simulink model "AbstractTwoVehicleModel"  (R2019b)
settings: Solver=VariableStepAuto  StartTime=0.0  StopTime=50  RelTol=1e-3
model workspace (MAT data in the model file):
  DOWN_TABLE = Simulink.Parameter
  DOWN_TABLE.Value = [0  2.2352  8.9408  15.6464; 0  2.2352  8.9408  15.6464; 0  2.2352  11.176  17.8816; 0  2.2352  13.4112  22.352; 0  13.4112  22.352  35.7632; 0  13.4112  22.352  35.7632]
  DOWN_TABLE.DataType = 'auto'
  DOWN_TABLE.Dimensions = [6 4]
  DOWN_TH_BP = Simulink.Parameter
  DOWN_TH_BP.Value = [0; 25; 35; 50; 90; 100]
  DOWN_TH_BP.DataType = 'auto'
  DOWN_TH_BP.Dimensions = [6 1]
  TWAIT = Simulink.Parameter
  TWAIT.Value = 2
  TWAIT.DataType = 'auto'
  TWAIT.Dimensions = [1 1]
  UP_TABLE = Simulink.Parameter
  UP_TABLE.Value = [4.4704  13.4112  22.352  447040; 4.4704  13.4112  22.352  447040; 6.7056  13.4112  22.352  447040; 10.28192  18.32864  26.8224  447040; 17.8816  31.2928  44.704  447040; 17.8816  31.2928  44.704  447040]
  UP_TABLE.DataType = 'auto'
  UP_TABLE.Dimensions = [6 4]
  UP_TH_BP = Simulink.Parameter
  UP_TH_BP.Value = [0; 25; 35; 50; 90; 100]
  UP_TH_BP.DataType = 'auto'
  UP_TH_BP.Dimensions = [6 1]
libraries: simulink x2, mpcadaslib x2
settings Model: Creator=qihan  LastModifiedBy=mustafa
settings SolverCC: ZeroCrossControl=DisableAll  ZeroCrossAlgorithm=Adaptive  DecoupledContinuousIntegration=on
settings DataIOCC: ReturnWorkspaceOutputsName=tpef60d72c_44c7_4a69_b2c5_cdb6ae33fc37
settings DebuggingCC: IgnoredZcDiagnostic=none
settings SFSimCC: CustomCodeUndefinedFunction=UseInterfaceOnly

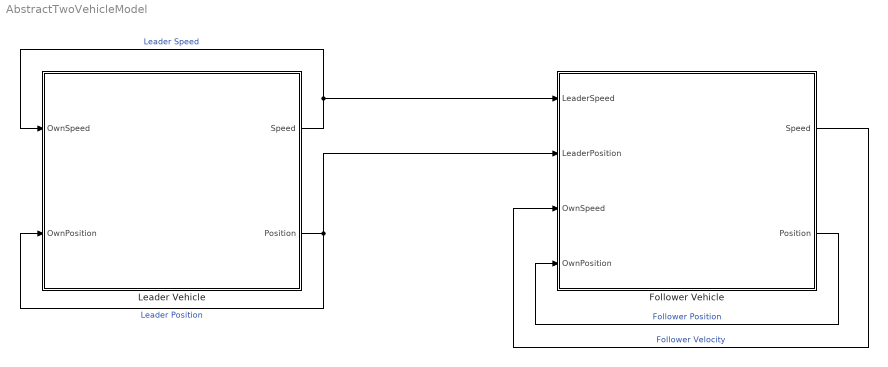
== system AbstractTwoVehicleModel ==
  Follower Vehicle : Subsystem  mask{InitPosition=0, FreeDriveSpeed=35, InitSpeed=45}
      mask prompts: InitPosition "Initial Position"; FreeDriveSpeed "FreeDrive Speed"; InitSpeed "Initial Speed"
      mask TypeOptions InitPosition: initial position/Value
      mask TypeOptions InitSpeed: initial Speed/Value
  Leader Vehicle : Subsystem  mask{InitPosition=100, FreeDriveSpeed=30, InitSpeed=30}
      mask prompts: InitPosition "Initial Position"; FreeDriveSpeed "FreeDrive Speed"; InitSpeed "Initial Speed"
      mask TypeOptions InitPosition: initial position/Value
      mask TypeOptions InitSpeed: initial Speed/Value
  wires:
  Leader Vehicle/1(Speed) -> Leader Vehicle/1(OwnSpeed), Follower Vehicle/1(LeaderSpeed)  "Leader Speed"
  Leader Vehicle/2(Position) -> Leader Vehicle/2(OwnPosition), Follower Vehicle/2(LeaderPosition)  "Leader Position"
  Follower Vehicle/1(Speed) -> Follower Vehicle/3(OwnSpeed)  "Follower Velocity"
  Follower Vehicle/2(Position) -> Follower Vehicle/4(OwnPosition)  "Follower Position"

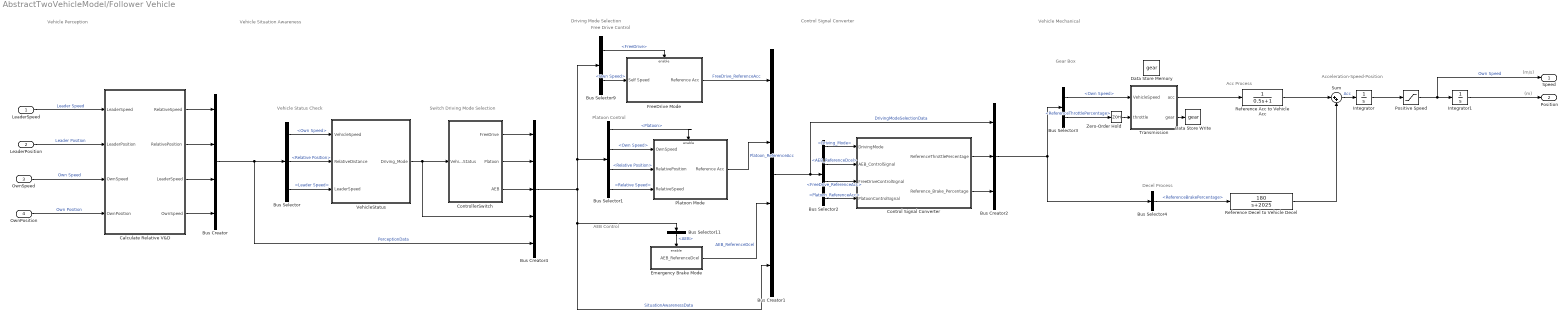
== system AbstractTwoVehicleModel/Follower Vehicle ==
  note: Acceleration-Speed-Position
  note: Vehicle Situation Awareness
  note: Driving Mode Selection
  note: Vehicle Mechanical
  note: AEB Control
  note: Free Drive Control
  note: Platoon Control
  note: Vehicle Status Check
  note: Acc Process
  note: (m)
  note: (m/s)
  note: Decel Process
  note: Vehicle Perception
  note: Switch Driving Mode Selection
  note: Control Signal Converter
  note: Gear Box
  LeaderSpeed : Inport
  LeaderPosition : Inport  Port=2
  OwnSpeed : Inport  Port=3
  OwnPosition : Inport  Port=4
  Bus Creator : BusCreator  Inputs=4
  Bus Creator1 : BusCreator  Inputs=4
  Bus Creator2 : BusCreator  Inputs=3
  Bus Creator4 : BusCreator  Inputs=5
  Bus Selector : BusSelector  OutputSignals=Own Speed,Relative Position,Leader Speed
  Bus Selector1 : BusSelector  OutputSignals=Platoon,PerceptionData.Own Speed,PerceptionData.Relative Position,PerceptionData.Relative Speed
  Bus Selector11 : BusSelector  OutputSignals=AEB
  Bus Selector2 : BusSelector  OutputSignals=SituationAwarenessData.Driving_Mode,AEB_ReferenceDcel,FreeDrive_ReferenceAcc,Platoon_ReferenceAcc
  Bus Selector3 : BusSelector  OutputSignals=DrivingModeSelectionData.SituationAwarenessData.PerceptionData.Own Speed,ReferenceThrottlePercentage
  Bus Selector4 : BusSelector  OutputSignals=ReferenceBrakePercentage
  Bus Selector9 : BusSelector  OutputSignals=FreeDrive,PerceptionData.Own Speed
  Calculate Relative V&D : Subsystem
  Control Signal Converter : Subsystem
  ControllerSwitch : Stateflow chart  BlockKeywords=__PRM__SERIALIZED__DATA__:Stateflow Chart,Stateflow Diagram  TreatAsAtomicUnit=on
  Data Store Memory : DataStoreMemory  DataStoreName=gear  ReadBeforeWriteMsg=warning  WriteAfterWriteMsg=warning  WriteAfterReadMsg=warning  ShowAdditionalParam=off
  Data Store Write : DataStoreWrite  DataStoreName=gear
  Emergency Brake Mode : Subsystem  TreatAsAtomicUnit=on
  FreeDrive Mode : Subsystem  TreatAsAtomicUnit=on
  Integrator : Integrator  InitialCondition=InitSpeed
  Integrator1 : Integrator  InitialCondition=InitPosition
  Platoon Mode : Subsystem  TreatAsAtomicUnit=on
  Positive Speed : Saturate  UpperLimit=inf  LowerLimit=0
  Reference Acc to Vehicle Acc : TransferFcn  Denominator=[0.5 1]
  Reference Decel to Vehicle Decel : TransferFcn  Numerator=[180]  Denominator=[1 2025]
  Sum : Sum  Inputs=|++
  Transmission : Stateflow chart  BlockKeywords=__PRM__SERIALIZED__DATA__:Stateflow Chart,Stateflow Diagram  TreatAsAtomicUnit=on
  VehicleStatus : Stateflow chart  BlockKeywords=__PRM__SERIALIZED__DATA__:Stateflow Chart,Stateflow Diagram  TreatAsAtomicUnit=on
  Zero-Order Hold : ZeroOrderHold  SampleTime=-1
  Speed : Outport  VectorParamsAs1DForOutWhenUnconnected=off
  Position : Outport  Port=2  VectorParamsAs1DForOutWhenUnconnected=off
  wires:
  Reference Acc to Vehicle Acc/1 -> Sum/1
  Reference Decel to Vehicle Decel/1 -> Sum/2
  Sum/1 -> Integrator/1  "Acc"
  Bus Selector/2 -> VehicleStatus/2(RelativeDistance)  "<Relative Position>"
  Integrator/1 -> Positive Speed/1
  Bus Selector/1 -> VehicleStatus/1(VehicleSpeed)  "<Own Speed>"
  Transmission/1(acc) -> Reference Acc to Vehicle Acc/1
  Bus Selector/3 -> VehicleStatus/3(LeaderSpeed)  "<Leader Speed>"
  FreeDrive Mode/1(Reference Acc) -> Bus Creator1/1  "FreeDrive_ReferenceAcc"
  Platoon Mode/1(Reference Acc) -> Bus Creator1/2  "Platoon_ReferenceAcc"
  Emergency Brake Mode/1(AEB_ReferenceDcel) -> Bus Creator1/3  "AEB_ReferenceDcel"
  Positive Speed/1 -> Speed/1, Integrator1/1  "Own Speed"
  Integrator1/1 -> Position/1
  LeaderSpeed/1 -> Calculate Relative V&D/1(LeaderSpeed)  "Leader Speed"
  LeaderPosition/1 -> Calculate Relative V&D/2(LeaderPosition)  "Leader Position"
  Bus Selector9/2 -> FreeDrive Mode/1(Self Speed)  "<Own Speed>"
  Bus Selector9/1 -> FreeDrive Mode/Enable  "<FreeDrive>"
  Bus Selector11/1 -> Emergency Brake Mode/Enable  "<AEB>"
  OwnSpeed/1 -> Calculate Relative V&D/3(OwnSpeed)  "Own Speed"
  OwnPosition/1 -> Calculate Relative V&D/4(OwnPosition)  "Own Position"
  VehicleStatus/1(Driving_Mode) -> Bus Creator4/4, ControllerSwitch/1(Vehicle_Status)
  Transmission/2(gear) -> Data Store Write/1
  Calculate Relative V&D/2(RelativePosition) -> Bus Creator/2
  Calculate Relative V&D/1(RelativeSpeed) -> Bus Creator/1
  Calculate Relative V&D/3("LeaderSpeed ") -> Bus Creator/3
  Calculate Relative V&D/4("OwnSpeed ") -> Bus Creator/4
  Bus Creator/1 -> Bus Creator4/5, Bus Selector/1  "PerceptionData"
  ControllerSwitch/1(FreeDrive) -> Bus Creator4/1
  ControllerSwitch/2(Platoon) -> Bus Creator4/2
  ControllerSwitch/3(AEB) -> Bus Creator4/3
  Bus Creator4/1 -> Bus Selector9/1, Bus Selector1/1, Bus Creator1/4, Bus Selector11/1  "SituationAwarenessData"
  Bus Selector1/1 -> Platoon Mode/Enable  "<Platoon>"
  Bus Selector1/2 -> Platoon Mode/1(OwnSpeed)  "<Own Speed>"
  Bus Selector1/3 -> Platoon Mode/2(RelativePosition)  "<Relative Position>"
  Bus Selector1/4 -> Platoon Mode/3(RelativeSpeed)  "<Relative Speed>"
  Bus Creator1/1 -> Bus Creator2/1, Bus Selector2/1  "DrivingModeSelectionData"
  Bus Selector2/1 -> Control Signal Converter/1(DrivingMode)  "<Driving_Mode>"
  Bus Selector2/2 -> Control Signal Converter/2(AEB_ControlSignal)  "<AEB_ReferenceDcel>"
  Bus Selector2/3 -> Control Signal Converter/3(FreeDriveControlSignal)  "<FreeDrive_ReferenceAcc>"
  Bus Selector2/4 -> Control Signal Converter/4(PlatoonControlSignal)  "<Platoon_ReferenceAcc>"
  Control Signal Converter/1(ReferenceThrottlePercentage) -> Bus Creator2/2
  Control Signal Converter/2(Reference_Brake_Percentage) -> Bus Creator2/3
  Bus Creator2/1 -> Bus Selector4/1, Bus Selector3/1
  Bus Selector3/1 -> Transmission/1(VehicleSpeed)  "<Own Speed>"
  Bus Selector3/2 -> Zero-Order Hold/1  "<ReferenceThrottlePercentage>"
  Bus Selector4/1 -> Reference Decel to Vehicle Decel/1  "<ReferenceBrakePercentage>"
  Zero-Order Hold/1 -> Transmission/2(throttle)

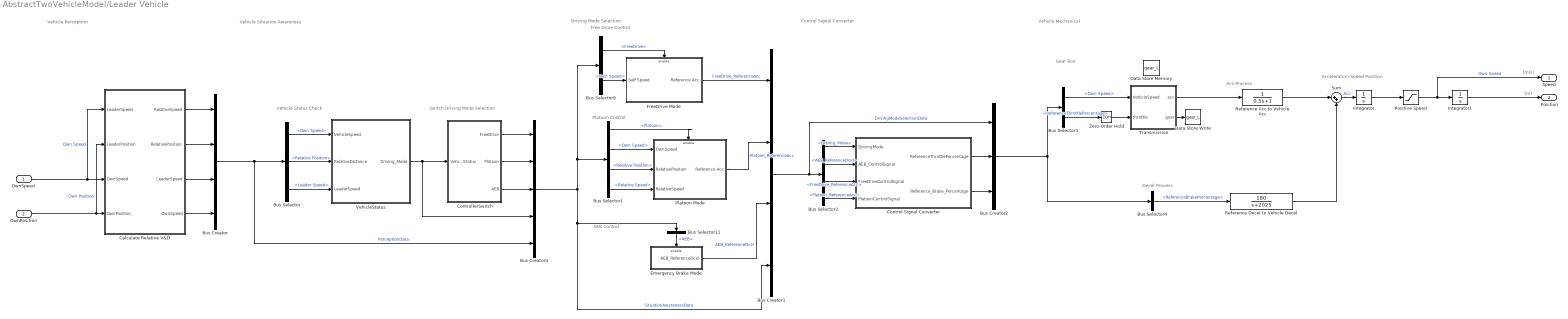
== system AbstractTwoVehicleModel/Leader Vehicle ==
  note: Acceleration-Speed-Position
  note: Vehicle Situation Awareness
  note: Driving Mode Selection
  note: Vehicle Mechanical
  note: AEB Control
  note: Free Drive Control
  note: Platoon Control
  note: Vehicle Status Check
  note: Acc Process
  note: (m)
  note: (m/s)
  note: Decel Process
  note: Vehicle Perception
  note: Switch Driving Mode Selection
  note: Control Signal Converter
  note: Gear Box
  OwnSpeed : Inport
  OwnPosition : Inport  Port=2
  Bus Creator : BusCreator  Inputs=4
  Bus Creator1 : BusCreator  Inputs=4
  Bus Creator2 : BusCreator  Inputs=3
  Bus Creator4 : BusCreator  Inputs=5
  Bus Selector : BusSelector  OutputSignals=Own Speed,Relative Position,Leader Speed
  Bus Selector1 : BusSelector  OutputSignals=Platoon,PerceptionData.Own Speed,PerceptionData.Relative Position,PerceptionData.Relative Speed
  Bus Selector11 : BusSelector  OutputSignals=AEB
  Bus Selector2 : BusSelector  OutputSignals=SituationAwarenessData.Driving_Mode,AEB_ReferenceDcel,FreeDrive_ReferenceAcc,Platoon_ReferenceAcc
  Bus Selector3 : BusSelector  OutputSignals=DrivingModeSelectionData.SituationAwarenessData.PerceptionData.Own Speed,ReferenceThrottlePercentage
  Bus Selector4 : BusSelector  OutputSignals=ReferenceBrakePercentage
  Bus Selector9 : BusSelector  OutputSignals=FreeDrive,PerceptionData.Own Speed
  Calculate Relative V&D : Subsystem
  Control Signal Converter : Subsystem
  ControllerSwitch : Stateflow chart  BlockKeywords=__PRM__SERIALIZED__DATA__:Stateflow Chart,Stateflow Diagram  TreatAsAtomicUnit=on
  Data Store Memory : DataStoreMemory  DataStoreName=gear_L  ReadBeforeWriteMsg=warning  WriteAfterWriteMsg=warning  WriteAfterReadMsg=warning  ShowAdditionalParam=off
  Data Store Write : DataStoreWrite  DataStoreName=gear_L
  Emergency Brake Mode : Subsystem  TreatAsAtomicUnit=on
  FreeDrive Mode : Subsystem  TreatAsAtomicUnit=on
  Integrator : Integrator  InitialCondition=InitSpeed
  Integrator1 : Integrator  InitialCondition=InitPosition
  Platoon Mode : Subsystem  TreatAsAtomicUnit=on
  Positive Speed : Saturate  UpperLimit=inf  LowerLimit=0
  Reference Acc to Vehicle Acc : TransferFcn  Denominator=[0.5 1]
  Reference Decel to Vehicle Decel : TransferFcn  Numerator=[180]  Denominator=[1 2025]
  Sum : Sum  Inputs=|++
  Transmission : Stateflow chart  BlockKeywords=__PRM__SERIALIZED__DATA__:Stateflow Chart,Stateflow Diagram  TreatAsAtomicUnit=on
  VehicleStatus : Stateflow chart  BlockKeywords=__PRM__SERIALIZED__DATA__:Stateflow Chart,Stateflow Diagram  TreatAsAtomicUnit=on
  Zero-Order Hold : ZeroOrderHold  SampleTime=-1
  Speed : Outport  VectorParamsAs1DForOutWhenUnconnected=off
  Position : Outport  Port=2  VectorParamsAs1DForOutWhenUnconnected=off
  wires:
  Reference Acc to Vehicle Acc/1 -> Sum/1
  Reference Decel to Vehicle Decel/1 -> Sum/2
  Sum/1 -> Integrator/1  "Acc"
  Bus Selector/2 -> VehicleStatus/2(RelativeDistance)  "<Relative Position>"
  Integrator/1 -> Positive Speed/1
  Bus Selector/1 -> VehicleStatus/1(VehicleSpeed)  "<Own Speed>"
  Transmission/1(acc) -> Reference Acc to Vehicle Acc/1
  Bus Selector/3 -> VehicleStatus/3(LeaderSpeed)  "<Leader Speed>"
  FreeDrive Mode/1(Reference Acc) -> Bus Creator1/1  "FreeDrive_ReferenceAcc"
  Platoon Mode/1(Reference Acc) -> Bus Creator1/2  "Platoon_ReferenceAcc"
  Emergency Brake Mode/1(AEB_ReferenceDcel) -> Bus Creator1/3  "AEB_ReferenceDcel"
  Positive Speed/1 -> Speed/1, Integrator1/1  "Own Speed"
  Integrator1/1 -> Position/1
  Bus Selector9/2 -> FreeDrive Mode/1(Self Speed)  "<Own Speed>"
  Bus Selector9/1 -> FreeDrive Mode/Enable  "<FreeDrive>"
  Bus Selector11/1 -> Emergency Brake Mode/Enable  "<AEB>"
  OwnSpeed/1 -> Calculate Relative V&D/1(LeaderSpeed), Calculate Relative V&D/3(OwnSpeed)  "Own Speed"
  OwnPosition/1 -> Calculate Relative V&D/2(LeaderPosition), Calculate Relative V&D/4(OwnPosition)  "Own Position"
  VehicleStatus/1(Driving_Mode) -> Bus Creator4/4, ControllerSwitch/1(Vehicle_Status)
  Transmission/2(gear) -> Data Store Write/1
  Calculate Relative V&D/2(RelativePosition) -> Bus Creator/2
  Calculate Relative V&D/1(RelativeSpeed) -> Bus Creator/1
  Calculate Relative V&D/3("LeaderSpeed ") -> Bus Creator/3
  Calculate Relative V&D/4("OwnSpeed ") -> Bus Creator/4
  Bus Creator/1 -> Bus Creator4/5, Bus Selector/1  "PerceptionData"
  ControllerSwitch/1(FreeDrive) -> Bus Creator4/1
  ControllerSwitch/2(Platoon) -> Bus Creator4/2
  ControllerSwitch/3(AEB) -> Bus Creator4/3
  Bus Creator4/1 -> Bus Selector9/1, Bus Selector1/1, Bus Creator1/4, Bus Selector11/1  "SituationAwarenessData"
  Bus Selector1/1 -> Platoon Mode/Enable  "<Platoon>"
  Bus Selector1/2 -> Platoon Mode/1(OwnSpeed)  "<Own Speed>"
  Bus Selector1/3 -> Platoon Mode/2(RelativePosition)  "<Relative Position>"
  Bus Selector1/4 -> Platoon Mode/3(RelativeSpeed)  "<Relative Speed>"
  Bus Creator1/1 -> Bus Creator2/1, Bus Selector2/1  "DrivingModeSelectionData"
  Bus Selector2/1 -> Control Signal Converter/1(DrivingMode)  "<Driving_Mode>"
  Bus Selector2/2 -> Control Signal Converter/2(AEB_ControlSignal)  "<AEB_ReferenceDcel>"
  Bus Selector2/3 -> Control Signal Converter/3(FreeDriveControlSignal)  "<FreeDrive_ReferenceAcc>"
  Bus Selector2/4 -> Control Signal Converter/4(PlatoonControlSignal)  "<Platoon_ReferenceAcc>"
  Control Signal Converter/1(ReferenceThrottlePercentage) -> Bus Creator2/2
  Control Signal Converter/2(Reference_Brake_Percentage) -> Bus Creator2/3
  Bus Creator2/1 -> Bus Selector4/1, Bus Selector3/1
  Bus Selector3/1 -> Transmission/1(VehicleSpeed)  "<Own Speed>"
  Bus Selector3/2 -> Zero-Order Hold/1  "<ReferenceThrottlePercentage>"
  Bus Selector4/1 -> Reference Decel to Vehicle Decel/1  "<ReferenceBrakePercentage>"
  Zero-Order Hold/1 -> Transmission/2(throttle)

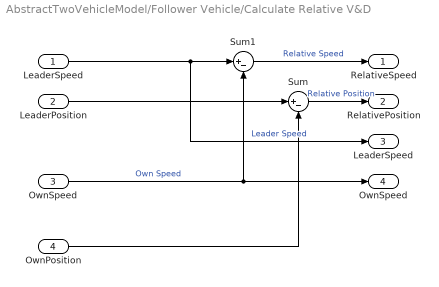
== system AbstractTwoVehicleModel/Follower Vehicle/Calculate Relative V&D ==
  LeaderSpeed : Inport
  LeaderPosition : Inport  Port=2
  OwnSpeed : Inport  Port=3
  OwnPosition : Inport  Port=4
  Sum : Sum  Inputs=|+-
  Sum1 : Sum  Inputs=|+-
  RelativeSpeed : Outport  VectorParamsAs1DForOutWhenUnconnected=off
  RelativePosition : Outport  Port=2  VectorParamsAs1DForOutWhenUnconnected=off
  "LeaderSpeed " : Outport  Port=3  VectorParamsAs1DForOutWhenUnconnected=off
  "OwnSpeed " : Outport  Port=4  VectorParamsAs1DForOutWhenUnconnected=off
  wires:
  Sum/1 -> RelativePosition/1  "Relative Position"
  LeaderPosition/1 -> Sum/1
  LeaderSpeed/1 -> "LeaderSpeed "/1, Sum1/1  "Leader Speed"
  OwnPosition/1 -> Sum/2
  Sum1/1 -> RelativeSpeed/1  "Relative Speed"
  OwnSpeed/1 -> "OwnSpeed "/1, Sum1/2  "Own Speed"

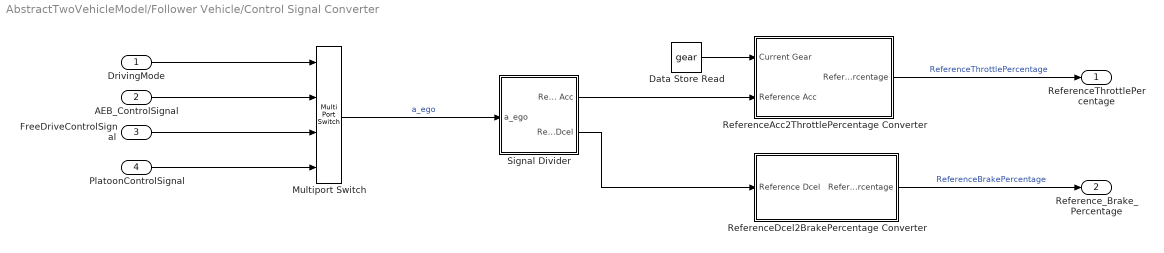
== system AbstractTwoVehicleModel/Follower Vehicle/Control Signal Converter ==
  DrivingMode : Inport
  AEB_ControlSignal : Inport  Port=2
  FreeDriveControlSignal : Inport  Port=3
  PlatoonControlSignal : Inport  Port=4
  Data Store Read : DataStoreRead  DataStoreName=gear
  Multiport Switch : MultiPortSwitch  DiagnosticForDefault=None
  ReferenceAcc2ThrottlePercentage Converter : Subsystem
  ReferenceDcel2BrakePercentage Converter : Subsystem
  Signal Divider : Subsystem
  ReferenceThrottlePercentage : Outport  VectorParamsAs1DForOutWhenUnconnected=off
  Reference_Brake_Percentage : Outport  Port=2  VectorParamsAs1DForOutWhenUnconnected=off
  wires:
  Signal Divider/1(Reference Acc) -> ReferenceAcc2ThrottlePercentage Converter/2(Reference Acc)
  ReferenceDcel2BrakePercentage Converter/1(Reference Brake Percentage) -> Reference_Brake_Percentage/1  "ReferenceBrakePercentage"
  Signal Divider/2(Reference Dcel) -> ReferenceDcel2BrakePercentage Converter/1(Reference Dcel)
  Multiport Switch/1 -> Signal Divider/1(a_ego)  "a_ego"
  Data Store Read/1 -> ReferenceAcc2ThrottlePercentage Converter/1(Current Gear)
  ReferenceAcc2ThrottlePercentage Converter/1(Reference Throttle Percentage) -> ReferenceThrottlePercentage/1  "ReferenceThrottlePercentage"
  DrivingMode/1 -> Multiport Switch/1
  AEB_ControlSignal/1 -> Multiport Switch/2
  FreeDriveControlSignal/1 -> Multiport Switch/3
  PlatoonControlSignal/1 -> Multiport Switch/4

== system AbstractTwoVehicleModel/Follower Vehicle/Emergency Brake Mode ==
  Enable : EnablePort
  Constant : Constant  Value=-10
  AEB_ReferenceDcel : Outport  OutputWhenDisabled=reset  InitialOutput=[0]  VectorParamsAs1DForOutWhenUnconnected=off
  wires:
  Constant/1 -> AEB_ReferenceDcel/1

== system AbstractTwoVehicleModel/Follower Vehicle/FreeDrive Mode ==
  Self Speed : Inport
  Enable : EnablePort  StatesWhenEnabling=reset
  FreeDrive Speed : Constant  Value=FreeDriveSpeed
  PID Controller1 : simulink/Continuous/PID Controller  Controller=PI  Form=Parallel  TimeDomain=Continuous-time  SampleTime=-1  IntegratorMethod=Forward Euler  FilterMethod=Forward Euler  ControllerParametersSource=internal  P=2.0341199375219  I=0.0356576460366845  D=2.08363010404189  UseFilter=on  N=233.214579742572  TunerSelectOption=Transfer Function Based (PID Tuner App)  ZeroCross=off  InitialConditionSource=internal  InitialConditionForIntegrator=0  InitialConditionForFilter=0  DifferentiatorICPrevScaledInput=0  ExternalReset=none  IgnoreLimit=on  TrackingMode=off  Kt=1  LimitOutput=on  UpperSaturationLimit=2  LowerSaturationLimit=-2  LinearizeAsGain=on  AntiWindupMode=clamping  Kb=1  POutMin=[]  POutMax=[]  IOutMin=[]  IOutMax=[]  DOutMin=[]  DOutMax=[]  NOutMin=[]  NOutMax=[]  SumOutMin=[]  SumOutMax=[]  SaturationOutMin=[]  SaturationOutMax=[]  PParamMin=[]  PParamMax=[]  IParamMin=[]  IParamMax=[]  DParamMin=[]  DParamMax=[]  NParamMin=[]  NParamMax=[]  KbParamMin=[]  KbParamMax=[]  KtParamMin=[]  KtParamMax=[]  KbOutMin=[]  KbOutMax=[]  KtOutMin=[]  KtOutMax=[]  IntegratorOutMin=[]  IntegratorOutMax=[]  FilterOutMin=[]  FilterOutMax=[]  SumI1OutMin=[]  SumI1OutMax=[]  SumI2OutMin=[]  SumI2OutMax=[]  SumI3OutMin=[]  SumI3OutMax=[]  SumI4OutMin=[]  SumI4OutMax=[]  SumDOutMin=[]  SumDOutMax=[]  DifferentiatorOutMin=[]  DifferentiatorOutMax=[]  FilterDiffOutCoefMin=[]  FilterDiffOutCoefMax=[]  ReciprocalOutMin=[]  ReciprocalOutMax=[]  SumDenOutMin=[]  SumDenOutMax=[]  SumNumOutMin=[]  SumNumOutMax=[]  DivideOutMin=[]  DivideOutMax=[]  IntegratorContinuousStateAttributes=''  IntegratorStateMustResolveToSignalObject=off  IntegratorRTWStateStorageClass=Auto  FilterContinuousStateAttributes=''  FilterStateMustResolveToSignalObject=off  FilterRTWStateStorageClass=Auto  ParallelPVariant=InternalParameters  IdealPVariant=Disabled  IVariant=InternalParameters  DVariant=Disabled  IntegratorVariant=Continuous  SatVariant=Enabled  AWVariant=ContClampingParallel  PCopyVariant=Disabled  TRVariant=Disabled  FdbkBlocksVariant=Forward  IdealPFdbkVariant=Disabled  SatFdbkVariant=Disabled  DerivativeFilterVariant=Disabled  NVariant=Disabled  NCopyVariant=Disabled_SignalSpec  FilterICVariant=Disabled  IntegratorICVariant=InternalICs  ExternalResetVariant=Disabled  TRSumVariant=Passthrough  SumFdbkVariant=Disabled  SumVariant=Sum_PI
  Sum16 : Sum  Inputs=|+-
  Reference Acc : Outport  OutputWhenDisabled=reset  InitialOutput=[0]  VectorParamsAs1DForOutWhenUnconnected=off
  wires:
  Self Speed/1 -> Sum16/2
  FreeDrive Speed/1 -> Sum16/1
  Sum16/1 -> PID Controller1/1
  PID Controller1/1 -> Reference Acc/1

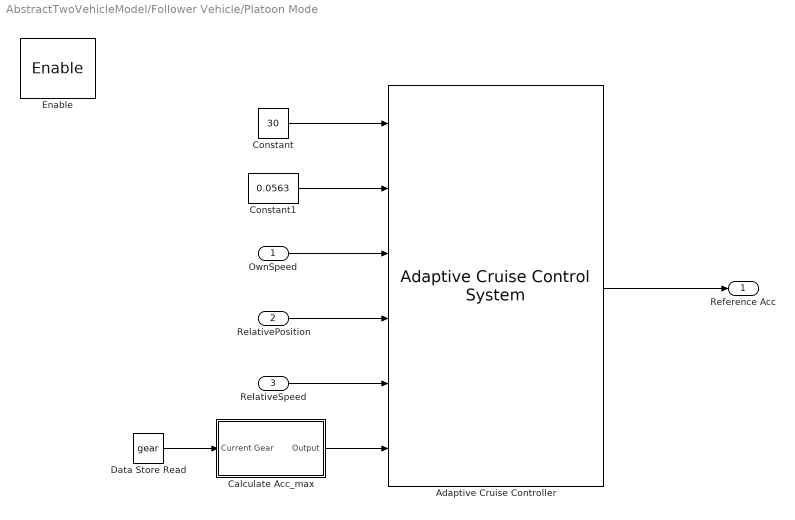
== system AbstractTwoVehicleModel/Follower Vehicle/Platoon Mode ==
  OwnSpeed : Inport
  RelativePosition : Inport  Port=2
  RelativeSpeed : Inport  Port=3
  Enable : EnablePort  StatesWhenEnabling=reset
  Adaptive Cruise Controller : mpcadaslib/Adaptive Cruise Control System  EgoModel=tf(1,[0.5,1,0])  InitialEgoVelocity=20  DefaultSpacing=10  MaxVelocity=50  MinAcceleration=-2  amin_ext=off  MaxAcceleration=2  amax_ext=on  Ts=0.1  PredictionHorizon=30  ControllerBehavior=0.260  suboptimal=off  maxiter=10  datatypeopt=double  optmode=off  trackmode=off
      settings: SourceProductName=Model Predictive Control Toolbox
  Calculate Acc_max : Subsystem
  Constant : Constant  Value=30
  Constant1 : Constant  Value=0.0563
  Data Store Read : DataStoreRead  DataStoreName=gear
  Reference Acc : Outport  OutputWhenDisabled=reset  InitialOutput=[0]  VectorParamsAs1DForOutWhenUnconnected=off
  wires:
  Constant/1 -> Adaptive Cruise Controller/1
  OwnSpeed/1 -> Adaptive Cruise Controller/3
  RelativePosition/1 -> Adaptive Cruise Controller/4
  RelativeSpeed/1 -> Adaptive Cruise Controller/5
  Adaptive Cruise Controller/1 -> Reference Acc/1
  Data Store Read/1 -> Calculate Acc_max/1(Current Gear)
  Calculate Acc_max/1(Output) -> Adaptive Cruise Controller/6
  Constant1/1 -> Adaptive Cruise Controller/2

== system AbstractTwoVehicleModel/Follower Vehicle/Transmission/ComputeThreshold ==
  note: Threshold Calculation
  gear : Inport  OutDataTypeStr=double  PortDimensions=1
  throttle : Inport  Port=2  OutDataTypeStr=double  PortDimensions=1
  f : TriggerPort  TriggerType=function-call  VariantControl=(inherit)
      settings: CopyFcn=Stateflow.SLINSF.SimulinkMan.removeBlockPreDeleteFcn  PreDeleteFcn=Stateflow.SLINSF.SimulinkMan.unsafePredeleteFcn
  InterpDown : Lookup_n-D  BreakpointsForDimension1=DOWN_TH_BP  BreakpointsForDimension2=[1:4]  Table=DOWN_TABLE  OutDataTypeStr=double  LockScale=on
  InterpUp : Lookup_n-D  BreakpointsForDimension1=UP_TH_BP  BreakpointsForDimension2=[1:4]  Table=UP_TABLE  OutDataTypeStr=double  LockScale=on
  down_th : Outport  VectorParamsAs1DForOutWhenUnconnected=off
  up_th : Outport  Port=2  VectorParamsAs1DForOutWhenUnconnected=off
  wires:
  throttle/1 -> InterpDown/1, InterpUp/1
  gear/1 -> InterpDown/2, InterpUp/2
  InterpDown/1 -> down_th/1
  InterpUp/1 -> up_th/1

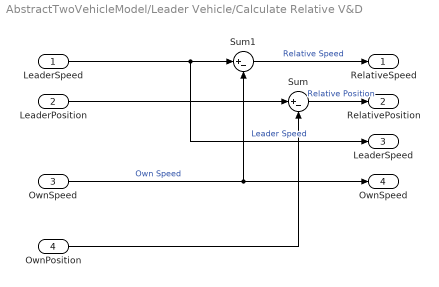
== system AbstractTwoVehicleModel/Leader Vehicle/Calculate Relative V&D ==
  LeaderSpeed : Inport
  LeaderPosition : Inport  Port=2
  OwnSpeed : Inport  Port=3
  OwnPosition : Inport  Port=4
  Sum : Sum  Inputs=|+-
  Sum1 : Sum  Inputs=|+-
  RelativeSpeed : Outport  VectorParamsAs1DForOutWhenUnconnected=off
  RelativePosition : Outport  Port=2  VectorParamsAs1DForOutWhenUnconnected=off
  "LeaderSpeed " : Outport  Port=3  VectorParamsAs1DForOutWhenUnconnected=off
  "OwnSpeed " : Outport  Port=4  VectorParamsAs1DForOutWhenUnconnected=off
  wires:
  Sum/1 -> RelativePosition/1  "Relative Position"
  LeaderPosition/1 -> Sum/1
  LeaderSpeed/1 -> "LeaderSpeed "/1, Sum1/1  "Leader Speed"
  OwnPosition/1 -> Sum/2
  Sum1/1 -> RelativeSpeed/1  "Relative Speed"
  OwnSpeed/1 -> "OwnSpeed "/1, Sum1/2  "Own Speed"

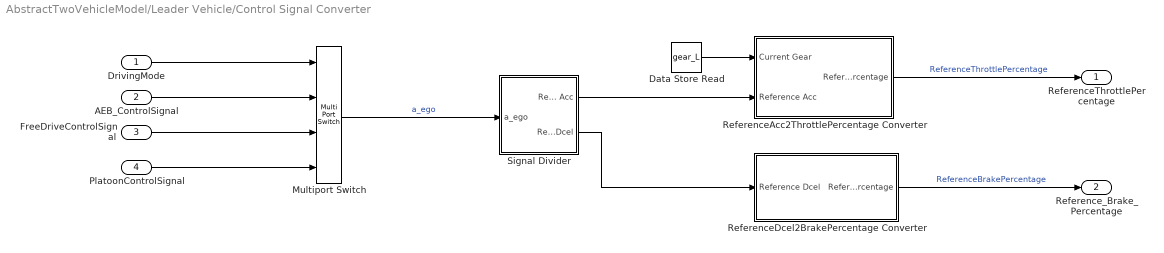
== system AbstractTwoVehicleModel/Leader Vehicle/Control Signal Converter ==
  DrivingMode : Inport
  AEB_ControlSignal : Inport  Port=2
  FreeDriveControlSignal : Inport  Port=3
  PlatoonControlSignal : Inport  Port=4
  Data Store Read : DataStoreRead  DataStoreName=gear_L
  Multiport Switch : MultiPortSwitch  DiagnosticForDefault=None
  ReferenceAcc2ThrottlePercentage Converter : Subsystem
  ReferenceDcel2BrakePercentage Converter : Subsystem
  Signal Divider : Subsystem
  ReferenceThrottlePercentage : Outport  VectorParamsAs1DForOutWhenUnconnected=off
  Reference_Brake_Percentage : Outport  Port=2  VectorParamsAs1DForOutWhenUnconnected=off
  wires:
  Signal Divider/1(Reference Acc) -> ReferenceAcc2ThrottlePercentage Converter/2(Reference Acc)
  ReferenceDcel2BrakePercentage Converter/1(Reference Brake Percentage) -> Reference_Brake_Percentage/1  "ReferenceBrakePercentage"
  Signal Divider/2(Reference Dcel) -> ReferenceDcel2BrakePercentage Converter/1(Reference Dcel)
  Multiport Switch/1 -> Signal Divider/1(a_ego)  "a_ego"
  Data Store Read/1 -> ReferenceAcc2ThrottlePercentage Converter/1(Current Gear)
  ReferenceAcc2ThrottlePercentage Converter/1(Reference Throttle Percentage) -> ReferenceThrottlePercentage/1  "ReferenceThrottlePercentage"
  DrivingMode/1 -> Multiport Switch/1
  AEB_ControlSignal/1 -> Multiport Switch/2
  FreeDriveControlSignal/1 -> Multiport Switch/3
  PlatoonControlSignal/1 -> Multiport Switch/4

== system AbstractTwoVehicleModel/Leader Vehicle/Emergency Brake Mode ==
  Enable : EnablePort
  Constant : Constant  Value=-10
  AEB_ReferenceDcel : Outport  OutputWhenDisabled=reset  InitialOutput=[0]  VectorParamsAs1DForOutWhenUnconnected=off
  wires:
  Constant/1 -> AEB_ReferenceDcel/1

== system AbstractTwoVehicleModel/Leader Vehicle/FreeDrive Mode ==
  Self Speed : Inport
  Enable : EnablePort  StatesWhenEnabling=reset
  FreeDrive Speed : Constant  Value=FreeDriveSpeed
  PID Controller1 : simulink/Continuous/PID Controller  Controller=PI  Form=Parallel  TimeDomain=Continuous-time  SampleTime=-1  IntegratorMethod=Forward Euler  FilterMethod=Forward Euler  ControllerParametersSource=internal  P=2.0341199375219  I=0.0356576460366845  D=2.08363010404189  UseFilter=on  N=233.214579742572  TunerSelectOption=Transfer Function Based (PID Tuner App)  ZeroCross=off  InitialConditionSource=internal  InitialConditionForIntegrator=0  InitialConditionForFilter=0  DifferentiatorICPrevScaledInput=0  ExternalReset=none  TrackingMode=off  Kt=1  LimitOutput=on  UpperSaturationLimit=2  LowerSaturationLimit=-3  LinearizeAsGain=on  AntiWindupMode=clamping  Kb=1  POutMin=[]  POutMax=[]  IOutMin=[]  IOutMax=[]  DOutMin=[]  DOutMax=[]  NOutMin=[]  NOutMax=[]  SumOutMin=[]  SumOutMax=[]  SaturationOutMin=[]  SaturationOutMax=[]  PParamMin=[]  PParamMax=[]  IParamMin=[]  IParamMax=[]  DParamMin=[]  DParamMax=[]  NParamMin=[]  NParamMax=[]  KbParamMin=[]  KbParamMax=[]  KtParamMin=[]  KtParamMax=[]  KbOutMin=[]  KbOutMax=[]  KtOutMin=[]  KtOutMax=[]  IntegratorOutMin=[]  IntegratorOutMax=[]  FilterOutMin=[]  FilterOutMax=[]  SumI1OutMin=[]  SumI1OutMax=[]  SumI2OutMin=[]  SumI2OutMax=[]  SumI3OutMin=[]  SumI3OutMax=[]  SumI4OutMin=[]  SumI4OutMax=[]  SumDOutMin=[]  SumDOutMax=[]  DifferentiatorOutMin=[]  DifferentiatorOutMax=[]  FilterDiffOutCoefMin=[]  FilterDiffOutCoefMax=[]  ReciprocalOutMin=[]  ReciprocalOutMax=[]  SumDenOutMin=[]  SumDenOutMax=[]  SumNumOutMin=[]  SumNumOutMax=[]  DivideOutMin=[]  DivideOutMax=[]  IntegratorContinuousStateAttributes=''  IntegratorStateMustResolveToSignalObject=off  IntegratorRTWStateStorageClass=Auto  FilterContinuousStateAttributes=''  FilterStateMustResolveToSignalObject=off  FilterRTWStateStorageClass=Auto  ParallelPVariant=InternalParameters  IdealPVariant=Disabled  IVariant=InternalParameters  DVariant=Disabled  IntegratorVariant=Continuous  SatVariant=Enabled  AWVariant=ContClampingParallel  PCopyVariant=Disabled  TRVariant=Disabled  FdbkBlocksVariant=Forward  IdealPFdbkVariant=Disabled  SatFdbkVariant=Disabled  DerivativeFilterVariant=Disabled  NVariant=Disabled  NCopyVariant=Disabled_SignalSpec  FilterICVariant=Disabled  IntegratorICVariant=InternalICs  ExternalResetVariant=Disabled  TRSumVariant=Passthrough  SumFdbkVariant=Disabled  SumVariant=Sum_PI
  Sum16 : Sum  Inputs=|+-
  Reference Acc : Outport  OutputWhenDisabled=reset  InitialOutput=[0]  VectorParamsAs1DForOutWhenUnconnected=off
  wires:
  Self Speed/1 -> Sum16/2
  FreeDrive Speed/1 -> Sum16/1
  Sum16/1 -> PID Controller1/1
  PID Controller1/1 -> Reference Acc/1

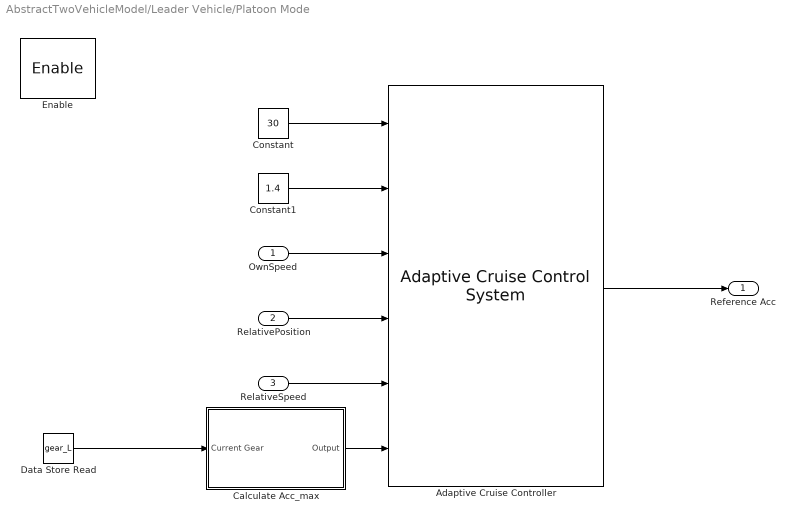
== system AbstractTwoVehicleModel/Leader Vehicle/Platoon Mode ==
  OwnSpeed : Inport
  RelativePosition : Inport  Port=2
  RelativeSpeed : Inport  Port=3
  Enable : EnablePort  StatesWhenEnabling=reset
  Adaptive Cruise Controller : mpcadaslib/Adaptive Cruise Control System  EgoModel=tf(1,[0.5,1,0])  InitialEgoVelocity=20  DefaultSpacing=10  MaxVelocity=50  MinAcceleration=-2  amin_ext=off  MaxAcceleration=2  amax_ext=on  Ts=0.1  PredictionHorizon=30  ControllerBehavior=0.5  suboptimal=off  maxiter=10  datatypeopt=double  optmode=off  trackmode=off
      settings: SourceProductName=Model Predictive Control Toolbox
  Calculate Acc_max : Subsystem
  Constant : Constant  Value=30
  Constant1 : Constant  Value=1.4
  Data Store Read : DataStoreRead  DataStoreName=gear_L
  Reference Acc : Outport  OutputWhenDisabled=reset  InitialOutput=[0]  VectorParamsAs1DForOutWhenUnconnected=off
  wires:
  Constant/1 -> Adaptive Cruise Controller/1
  OwnSpeed/1 -> Adaptive Cruise Controller/3
  RelativePosition/1 -> Adaptive Cruise Controller/4
  RelativeSpeed/1 -> Adaptive Cruise Controller/5
  Adaptive Cruise Controller/1 -> Reference Acc/1
  Constant1/1 -> Adaptive Cruise Controller/2
  Data Store Read/1 -> Calculate Acc_max/1(Current Gear)
  Calculate Acc_max/1(Output) -> Adaptive Cruise Controller/6

== system AbstractTwoVehicleModel/Leader Vehicle/Transmission/ComputeThreshold ==
  note: Threshold Calculation
  gear : Inport  OutDataTypeStr=double  PortDimensions=1
  throttle : Inport  Port=2  OutDataTypeStr=double  PortDimensions=1
  f : TriggerPort  TriggerType=function-call  VariantControl=(inherit)
      settings: CopyFcn=Stateflow.SLINSF.SimulinkMan.removeBlockPreDeleteFcn  PreDeleteFcn=Stateflow.SLINSF.SimulinkMan.unsafePredeleteFcn
  InterpDown : Lookup_n-D  BreakpointsForDimension1=DOWN_TH_BP  BreakpointsForDimension2=[1:4]  Table=DOWN_TABLE  OutDataTypeStr=double  LockScale=on
  InterpUp : Lookup_n-D  BreakpointsForDimension1=UP_TH_BP  BreakpointsForDimension2=[1:4]  Table=UP_TABLE  OutDataTypeStr=double  LockScale=on
  down_th : Outport  VectorParamsAs1DForOutWhenUnconnected=off
  up_th : Outport  Port=2  VectorParamsAs1DForOutWhenUnconnected=off
  wires:
  throttle/1 -> InterpDown/1, InterpUp/1
  gear/1 -> InterpDown/2, InterpUp/2
  InterpDown/1 -> down_th/1
  InterpUp/1 -> up_th/1

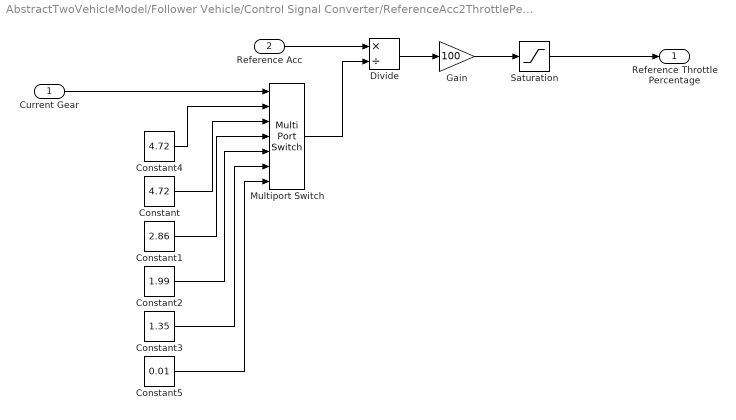
== system AbstractTwoVehicleModel/Follower Vehicle/Control Signal Converter/ReferenceAcc2ThrottlePercentage Converter ==
  Current Gear : Inport
  Reference Acc : Inport  Port=2
  Constant : Constant  Value=4.72
  Constant1 : Constant  Value=2.86
  Constant2 : Constant  Value=1.99
  Constant3 : Constant  Value=1.35
  Constant4 : Constant  Value=4.72
  Constant5 : Constant  Value=0.01
  Divide : Product  Inputs=*/
  Gain : Gain  Gain=100
  Multiport Switch : MultiPortSwitch  DataPortOrder=Zero-based contiguous  Inputs=6  zeroidx=on
  Saturation : Saturate  UpperLimit=100  LowerLimit=0  ZeroCross=off
  Reference Throttle Percentage : Outport  VectorParamsAs1DForOutWhenUnconnected=off
  wires:
  Multiport Switch/1 -> Divide/2
  Constant1/1 -> Multiport Switch/4
  Constant5/1 -> Multiport Switch/7
  Constant3/1 -> Multiport Switch/6
  Reference Acc/1 -> Divide/1
  Constant/1 -> Multiport Switch/3
  Constant4/1 -> Multiport Switch/2
  Constant2/1 -> Multiport Switch/5
  Current Gear/1 -> Multiport Switch/1
  Divide/1 -> Gain/1
  Gain/1 -> Saturation/1
  Saturation/1 -> Reference Throttle Percentage/1

== system AbstractTwoVehicleModel/Follower Vehicle/Control Signal Converter/ReferenceDcel2BrakePercentage Converter ==
  Reference Dcel : Inport
  Constant : Constant  Value=3
  Divide : Product  Inputs=*/
  Gain : Gain  Gain=100
  Saturation : Saturate  UpperLimit=0  LowerLimit=-100
  Reference Brake Percentage : Outport  VectorParamsAs1DForOutWhenUnconnected=off
  wires:
  Reference Dcel/1 -> Divide/1
  Divide/1 -> Gain/1
  Gain/1 -> Saturation/1
  Saturation/1 -> Reference Brake Percentage/1
  Constant/1 -> Divide/2

== system AbstractTwoVehicleModel/Follower Vehicle/Control Signal Converter/Signal Divider ==
  a_ego : Inport
  Constant2 : Constant  Value=0
  Switch : Switch  Criteria=u2 > Threshold
  Switch1 : Switch  Criteria=u2 > Threshold
  Reference Acc : Outport  VectorParamsAs1DForOutWhenUnconnected=off
  Reference Dcel : Outport  Port=2  VectorParamsAs1DForOutWhenUnconnected=off
  wires:
  Constant2/1 -> Switch1/1, Switch/3
  a_ego/1 -> Switch/1, Switch/2, Switch1/2, Switch1/3
  Switch1/1 -> Reference Dcel/1
  Switch/1 -> Reference Acc/1

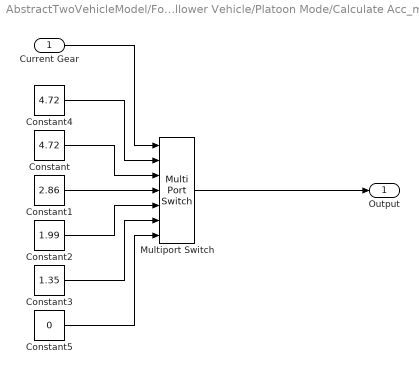
== system AbstractTwoVehicleModel/Follower Vehicle/Platoon Mode/Calculate Acc_max ==
  Current Gear : Inport
  Constant : Constant  Value=4.72
  Constant1 : Constant  Value=2.86
  Constant2 : Constant  Value=1.99
  Constant3 : Constant  Value=1.35
  Constant4 : Constant  Value=4.72
  Constant5 : Constant  Value=0
  Multiport Switch : MultiPortSwitch  DataPortOrder=Zero-based contiguous  Inputs=6  DiagnosticForDefault=None  zeroidx=on
  Output : Outport  VectorParamsAs1DForOutWhenUnconnected=off
  wires:
  Constant1/1 -> Multiport Switch/4
  Constant5/1 -> Multiport Switch/7
  Constant3/1 -> Multiport Switch/6
  Current Gear/1 -> Multiport Switch/1
  Constant/1 -> Multiport Switch/3
  Constant4/1 -> Multiport Switch/2
  Multiport Switch/1 -> Output/1
  Constant2/1 -> Multiport Switch/5

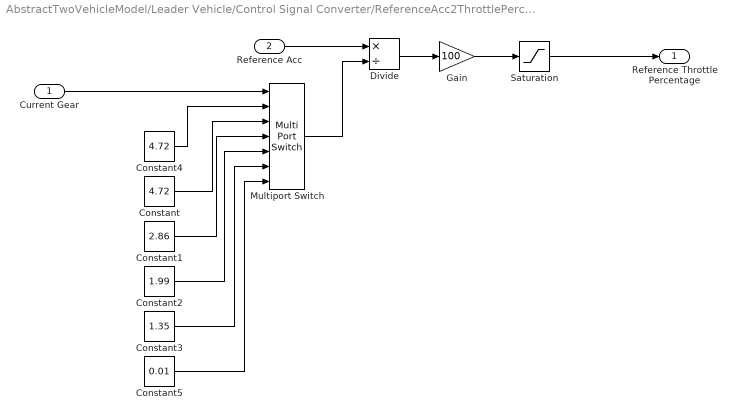
== system AbstractTwoVehicleModel/Leader Vehicle/Control Signal Converter/ReferenceAcc2ThrottlePercentage Converter ==
  Current Gear : Inport
  Reference Acc : Inport  Port=2
  Constant : Constant  Value=4.72
  Constant1 : Constant  Value=2.86
  Constant2 : Constant  Value=1.99
  Constant3 : Constant  Value=1.35
  Constant4 : Constant  Value=4.72
  Constant5 : Constant  Value=0.01
  Divide : Product  Inputs=*/
  Gain : Gain  Gain=100
  Multiport Switch : MultiPortSwitch  DataPortOrder=Zero-based contiguous  Inputs=6  zeroidx=on
  Saturation : Saturate  UpperLimit=100  LowerLimit=0  ZeroCross=off
  Reference Throttle Percentage : Outport  VectorParamsAs1DForOutWhenUnconnected=off
  wires:
  Multiport Switch/1 -> Divide/2
  Constant1/1 -> Multiport Switch/4
  Constant5/1 -> Multiport Switch/7
  Constant3/1 -> Multiport Switch/6
  Reference Acc/1 -> Divide/1
  Constant/1 -> Multiport Switch/3
  Constant4/1 -> Multiport Switch/2
  Constant2/1 -> Multiport Switch/5
  Current Gear/1 -> Multiport Switch/1
  Divide/1 -> Gain/1
  Gain/1 -> Saturation/1
  Saturation/1 -> Reference Throttle Percentage/1

== system AbstractTwoVehicleModel/Leader Vehicle/Control Signal Converter/ReferenceDcel2BrakePercentage Converter ==
  Reference Dcel : Inport
  Constant : Constant  Value=3
  Divide : Product  Inputs=*/
  Gain : Gain  Gain=100
  Saturation : Saturate  UpperLimit=0  LowerLimit=-100
  Reference Brake Percentage : Outport  VectorParamsAs1DForOutWhenUnconnected=off
  wires:
  Reference Dcel/1 -> Divide/1
  Divide/1 -> Gain/1
  Gain/1 -> Saturation/1
  Saturation/1 -> Reference Brake Percentage/1
  Constant/1 -> Divide/2

== system AbstractTwoVehicleModel/Leader Vehicle/Control Signal Converter/Signal Divider ==
  a_ego : Inport
  Constant2 : Constant  Value=0
  Switch : Switch  Criteria=u2 > Threshold
  Switch1 : Switch  Criteria=u2 > Threshold
  Reference Acc : Outport  VectorParamsAs1DForOutWhenUnconnected=off
  Reference Dcel : Outport  Port=2  VectorParamsAs1DForOutWhenUnconnected=off
  wires:
  Constant2/1 -> Switch1/1, Switch/3
  a_ego/1 -> Switch/1, Switch/2, Switch1/2, Switch1/3
  Switch1/1 -> Reference Dcel/1
  Switch/1 -> Reference Acc/1

== system AbstractTwoVehicleModel/Leader Vehicle/Platoon Mode/Calculate Acc_max ==
  Current Gear : Inport
  Constant : Constant  Value=4.72
  Constant1 : Constant  Value=2.86
  Constant2 : Constant  Value=1.99
  Constant3 : Constant  Value=1.35
  Constant4 : Constant  Value=4.72
  Constant5 : Constant  Value=0
  Multiport Switch : MultiPortSwitch  DataPortOrder=Zero-based contiguous  Inputs=6  DiagnosticForDefault=None  zeroidx=on
  Output : Outport  VectorParamsAs1DForOutWhenUnconnected=off
  wires:
  Constant1/1 -> Multiport Switch/4
  Constant5/1 -> Multiport Switch/7
  Constant3/1 -> Multiport Switch/6
  Current Gear/1 -> Multiport Switch/1
  Constant/1 -> Multiport Switch/3
  Constant4/1 -> Multiport Switch/2
  Multiport Switch/1 -> Output/1
  Constant2/1 -> Multiport Switch/5

== stateflow chart AbstractTwoVehicleModel/Leader Vehicle/ControllerSwitch ==
  state Platoon_Controller
    entry:
    Platoon=1;
    FreeDrive=0;
    AEB=0;
  state Choose_Controller
    entry:
    Platoon=0;
    FreeDrive=0;
    AEB=0;
  state FreeDrive_Controller
    entry:
    Platoon=0;
    FreeDrive=1;
    AEB=0;
  state AEB
    entry:
    Platoon=0;
    FreeDrive=0;
    AEB=1;
  (default) -> Choose_Controller
  Choose_Controller -> Platoon_Controller [order 2] : [Vehicle_Status==3]
  FreeDrive_Controller -> Platoon_Controller [order 1] : [Vehicle_Status==3]
  Platoon_Controller -> FreeDrive_Controller [order 2] : [Vehicle_Status==2]
  Platoon_Controller -> AEB [order 1] : [Vehicle_Status==1]
  AEB -> Platoon_Controller [order 2] : [Vehicle_Status==3]
  Choose_Controller -> FreeDrive_Controller [order 1] : [Vehicle_Status==2]
  Choose_Controller -> AEB [order 3] : [Vehicle_Status==1]
  FreeDrive_Controller -> AEB [order 2] : [Vehicle_Status==1]
  AEB -> FreeDrive_Controller [order 1] : [Vehicle_Status==2]
  data: FreeDrive output; Platoon output; Vehicle_Status input; AEB output

== stateflow chart AbstractTwoVehicleModel/Follower Vehicle/ControllerSwitch ==
  state Platoon_Controller
    entry:
    Platoon=1;
    FreeDrive=0;
    AEB=0;
  state Choose_Controller
    entry:
    Platoon=0;
    FreeDrive=0;
    AEB=0;
  state FreeDrive_Controller
    entry:
    Platoon=0;
    FreeDrive=1;
    AEB=0;
  state AEB
    entry:
    Platoon=0;
    FreeDrive=0;
    AEB=1;
  (default) -> Choose_Controller
  Choose_Controller -> Platoon_Controller [order 2] : [Vehicle_Status==3]
  FreeDrive_Controller -> Platoon_Controller [order 1] : [Vehicle_Status==3]
  Platoon_Controller -> FreeDrive_Controller [order 2] : [Vehicle_Status==2]
  Platoon_Controller -> AEB [order 1] : [Vehicle_Status==1]
  AEB -> Platoon_Controller [order 2] : [Vehicle_Status==3]
  Choose_Controller -> FreeDrive_Controller [order 1] : [Vehicle_Status==2]
  Choose_Controller -> AEB [order 3] : [Vehicle_Status==1]
  FreeDrive_Controller -> AEB [order 2] : [Vehicle_Status==1]
  AEB -> FreeDrive_Controller [order 1] : [Vehicle_Status==2]
  data: FreeDrive output; Platoon output; Vehicle_Status input; AEB output

== stateflow chart AbstractTwoVehicleModel/Follower Vehicle/Transmission ==
  state gear_state [parallel]
    settings: executionOrder=1
    state Check
      entry:
      gear = 0;
    state first
      gear = 1;
      acc=throttle*0.0472;
    state second
      gear = 2;
      acc=throttle*0.0286;
    state third
      gear = 3;
      acc=throttle*0.0199;
    state fourth
      gear = 4;
      acc=throttle*0.0135;
    state SpeedLimit
      entry:
      gear = 5;
      acc = 0;
    Check -> fourth [order 1] : [30<=VehicleSpeed]
    Check -> first [order 4] : [(0<=VehicleSpeed)&&(VehicleSpeed<10)]
    Check -> second [order 3] : [(10<=VehicleSpeed)&&(VehicleSpeed<20)]
    Check -> third [order 2] : [(20<=VehicleSpeed)&&(VehicleSpeed<30)]
    second -> third [order 1] : UP
    SpeedLimit -> fourth : [VehicleSpeed<60]
    fourth -> third [order 1] : DOWN
    first -> second : UP
    fourth -> SpeedLimit [order 2] : [VehicleSpeed>=60]
    second -> first [order 2] : DOWN
    third -> second [order 2] : DOWN
    third -> fourth [order 1] : UP
  state selection_state [parallel]
    during:
    [down_th, up_th] = ComputeThreshold(gear,throttle);
    settings: executionOrder=2
    state steady_state
    state upshifting
    state downshifting
    (default) -> steady_state
    steady_state -> upshifting [order 1] : [VehicleSpeed > up_th]
    steady_state -> downshifting [order 2] : [VehicleSpeed < down_th]
    downshifting -> steady_state [order 2] : [VehicleSpeed > down_th]
    downshifting -> steady_state [order 1] : after(TWAIT,tick)
        | [VehicleSpeed <= down_th]
        | {gear_state.DOWN}
    upshifting -> steady_state [order 1] : after(TWAIT,tick)
        | [VehicleSpeed >= up_th]
        | {gear_state.UP}
    upshifting -> steady_state [order 2] : [VehicleSpeed < up_th]
  state [down_th,up_th] = ComputeThreshold(gear,throttle) [function]
  (default) -> Check
  data: gear function_input double size=1; throttle function_input double size=1; down_th function_output; up_th function_output; VehicleSpeed input; throttle input; acc output; up_th local; down_th local; TWAIT parameter; gear output
  events: DOWN local EITHER_EDGE_EVENT; UP local EITHER_EDGE_EVENT

== stateflow chart AbstractTwoVehicleModel/Leader Vehicle/Transmission ==
  state gear_state [parallel]
    settings: executionOrder=1
    state Check
      entry:
      gear = 0;
    state first
      gear = 1;
      acc=throttle*0.0472;
    state second
      gear = 2;
      acc=throttle*0.0286;
    state third
      gear = 3;
      acc=throttle*0.0199;
    state fourth
      gear = 4;
      acc=throttle*0.0135;
    state SpeedLimit
      entry:
      gear = 5;
      acc = 0;
    Check -> fourth [order 1] : [30<=VehicleSpeed]
    Check -> first [order 4] : [(0<=VehicleSpeed)&&(VehicleSpeed<10)]
    Check -> second [order 3] : [(10<=VehicleSpeed)&&(VehicleSpeed<20)]
    Check -> third [order 2] : [(20<=VehicleSpeed)&&(VehicleSpeed<30)]
    second -> third [order 1] : UP
    SpeedLimit -> fourth : [VehicleSpeed<60]
    fourth -> third [order 1] : DOWN
    first -> second : UP
    fourth -> SpeedLimit [order 2] : [VehicleSpeed>=60]
    second -> first [order 2] : DOWN
    third -> second [order 2] : DOWN
    third -> fourth [order 1] : UP
  state selection_state [parallel]
    during:
    [down_th, up_th] = ComputeThreshold(gear,throttle);
    settings: executionOrder=2
    state steady_state
    state upshifting
    state downshifting
    (default) -> steady_state
    steady_state -> upshifting [order 1] : [VehicleSpeed > up_th]
    steady_state -> downshifting [order 2] : [VehicleSpeed < down_th]
    downshifting -> steady_state [order 2] : [VehicleSpeed > down_th]
    downshifting -> steady_state [order 1] : after(TWAIT,tick)
        | [VehicleSpeed <= down_th]
        | {gear_state.DOWN}
    upshifting -> steady_state [order 1] : after(TWAIT,tick)
        | [VehicleSpeed >= up_th]
        | {gear_state.UP}
    upshifting -> steady_state [order 2] : [VehicleSpeed < up_th]
  state [down_th,up_th] = ComputeThreshold(gear,throttle) [function]
  (default) -> Check
  data: gear function_input double size=1; throttle function_input double size=1; down_th function_output; up_th function_output; VehicleSpeed input; throttle input; acc output; up_th local; down_th local; TWAIT parameter; gear output
  events: DOWN local EITHER_EDGE_EVENT; UP local EITHER_EDGE_EVENT

== stateflow chart AbstractTwoVehicleModel/Leader Vehicle/VehicleStatus ==
  state Vehicle_FreeDrive
    entry:
    Driving_Mode=2;
  state Mode_Check
    entry:
    Driving_Mode=0;
  state Vehicle_AEB
    entry:
    Driving_Mode=1;
  state Vehicle_Platooning
    entry:
    Driving_Mode=3;
  (default) -> Mode_Check
  Mode_Check -> Vehicle_FreeDrive [order 2] : [RelativeDistance>200]
  Vehicle_FreeDrive -> Vehicle_Platooning [order 2] : [(RelativeDistance<=200)&&(RelativeDistance>(get_SD(VehicleSpeed,LeaderSpeed)))]
  Vehicle_Platooning -> Vehicle_FreeDrive [order 1] : [RelativeDistance>200]
  Vehicle_FreeDrive -> Vehicle_AEB [order 1] : [(RelativeDistance<get_SD(VehicleSpeed,LeaderSpeed))]
  Vehicle_AEB -> Vehicle_FreeDrive [order 1] : [RelativeDistance>200]
  Mode_Check -> Vehicle_Platooning [order 1] : [(RelativeDistance<=200)&&(RelativeDistance>(get_SD(VehicleSpeed,LeaderSpeed)))]
  Mode_Check -> Vehicle_AEB [order 3] : [RelativeDistance<get_SD(VehicleSpeed,LeaderSpeed)]
  Vehicle_AEB -> Vehicle_Platooning [order 2] : [(RelativeDistance>(get_SD(VehicleSpeed,LeaderSpeed)))&&(RelativeDistance<200)]
  Vehicle_Platooning -> Vehicle_AEB [order 2] : [(RelativeDistance<get_SD(VehicleSpeed,LeaderSpeed))]
  data: x1 function_input; x2 function_input; SD function_output; VehicleSpeed input; throttle local; RelativeDistance input; LeaderSpeed input; Driving_Mode output
  function SD=get_SD(x1,x2):
    | function SD=get_SD(x1,x2)
    | SD=(x1-x2)^2*0.0563+2;

== stateflow chart AbstractTwoVehicleModel/Follower Vehicle/VehicleStatus ==
  state Vehicle_FreeDrive
    entry:
    Driving_Mode=2;
  state Mode_Check
    entry:
    Driving_Mode=0;
  state Vehicle_AEB
    entry:
    Driving_Mode=1;
  state Vehicle_Platooning
    entry:
    Driving_Mode=3;
  (default) -> Mode_Check
  Mode_Check -> Vehicle_FreeDrive [order 2] : [RelativeDistance>200]
  Vehicle_FreeDrive -> Vehicle_Platooning [order 2] : [(RelativeDistance<=200)&&(RelativeDistance>(get_SD(VehicleSpeed,LeaderSpeed)))]
  Vehicle_Platooning -> Vehicle_FreeDrive [order 1] : [RelativeDistance>200]
  Vehicle_FreeDrive -> Vehicle_AEB [order 1] : [(RelativeDistance<get_SD(VehicleSpeed,LeaderSpeed))]
  Vehicle_AEB -> Vehicle_FreeDrive [order 1] : [RelativeDistance>200]
  Mode_Check -> Vehicle_Platooning [order 1] : [(RelativeDistance<=200)&&(RelativeDistance>(get_SD(VehicleSpeed,LeaderSpeed)))]
  Mode_Check -> Vehicle_AEB [order 3] : [RelativeDistance<get_SD(VehicleSpeed,LeaderSpeed)]
  Vehicle_AEB -> Vehicle_Platooning [order 2] : [(RelativeDistance>(get_SD(VehicleSpeed,LeaderSpeed)))&&(RelativeDistance<200)]
  Vehicle_Platooning -> Vehicle_AEB [order 2] : [(RelativeDistance<get_SD(VehicleSpeed,LeaderSpeed))]
  data: x1 function_input; x2 function_input; SD function_output; VehicleSpeed input; throttle local; RelativeDistance input; LeaderSpeed input; Driving_Mode output
  function SD=get_SD(x1,x2):
    | function SD=get_SD(x1,x2)
    | SD=(x1-x2)^2*0.0563+2;
